simulink model "Simulink_Differentialgleichung"  (R2017b)
settings: Solver=VariableStepAuto  StartTime=0.0  StopTime=120  MaxStep=0.002  RelTol=1e-3
settings Model: Creator=aby032  LastModifiedBy=aby032

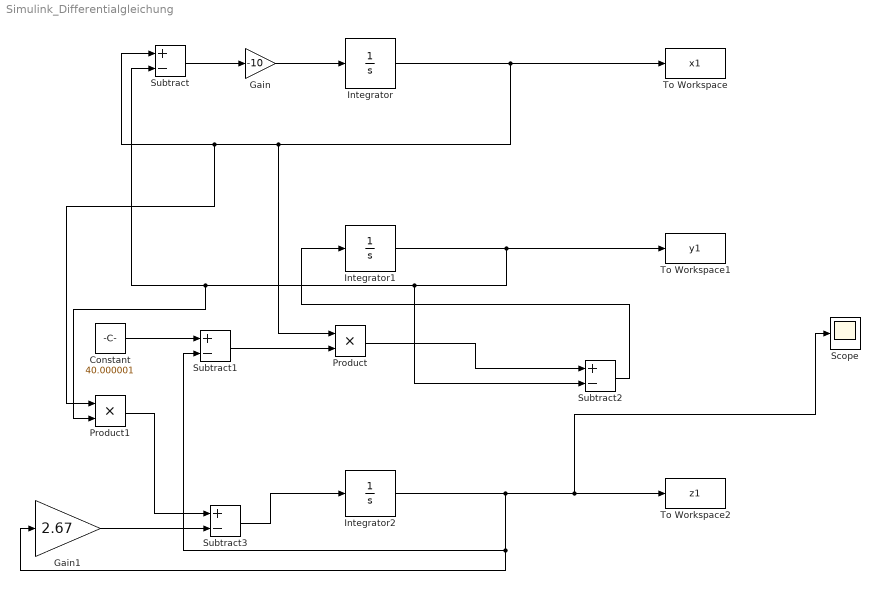
== system Simulink_Differentialgleichung ==
  Constant : Constant  Value=40.000001
  Gain : Gain  Gain=-10
  Gain1 : Gain  Gain=2.67
  Integrator : Integrator  InitialCondition=0.01
  Integrator1 : Integrator  InitialCondition=0.01
  Integrator2 : Integrator  InitialCondition=0.0
  Product : Product
  Product1 : Product
  Scope : Scope
  Subtract{,1..3} (4 alike) : Sum  Inputs=+-
  To Workspace : ToWorkspace  VariableName=x1  SampleTime=-1
  To Workspace1 : ToWorkspace  VariableName=y1  SampleTime=-1
  To Workspace2 : ToWorkspace  VariableName=z1  SampleTime=-1
  wires:
  Subtract/1 -> Gain/1
  Gain/1 -> Integrator/1
  Integrator1/1 -> Subtract2/2, Product1/2, Subtract/2, To Workspace1/1
  Integrator2/1 -> Gain1/1, Subtract1/2, Scope/1, To Workspace2/1
  Constant/1 -> Subtract1/1
  Subtract1/1 -> Product/2
  Product/1 -> Subtract2/1
  Subtract2/1 -> Integrator1/1
  Product1/1 -> Subtract3/1
  Gain1/1 -> Subtract3/2
  Subtract3/1 -> Integrator2/1
  Integrator/1 -> Product/1, Product1/1, Subtract/1, To Workspace/1
